simulink model "ex_2_20_1_simul"  (R2025a)
settings: Solver=VariableStepAuto  StartTime=0.0  StopTime=10.0  MaxStep=0.01  RelTol=1e-3
libraries: dspsrcs4 x1
settings Model: Creator=konstantin  LastModifiedBy=konstantin

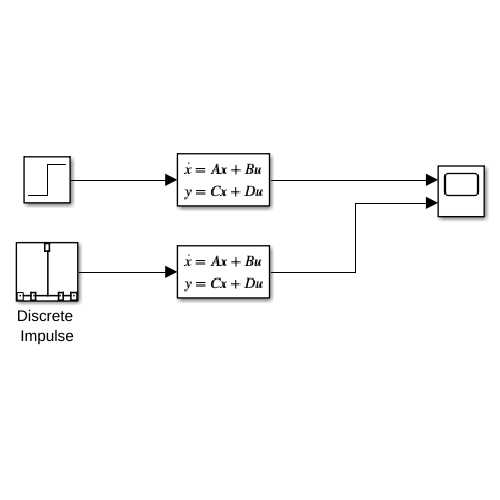
[thumbnail: Simulink's stored preview of the top-level diagram]
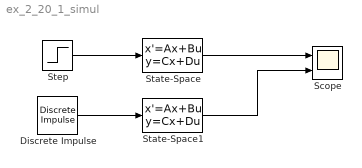
== system ex_2_20_1_simul ==
  Discrete Impulse : dspsrcs4/Discrete  Impulse  Delay=1  SampleTime=1  FrameSample=1  OutputFrames=off  dataType=double  isSigned=on  wordLen=16  udDataType=sfix(16)  fracBitsMode=Best precision  numFracBits=15  OutDataTypeStr=double  LastOutDataTypeStr=double
  Scope : Scope  NumInputPorts=2
      settings: ActiveDisplayYMinimum=-0.24999998857845496  ActiveDisplayYMaximum=2.2499998972060951
  State-Space : StateSpace  A=[-5, -6; 1, 0]  B=[1; 0]  C=[0, 12]  D=0  InitialCondition=0
  State-Space1 : StateSpace  A=[-5, -6; 1, 0]  B=[1; 0]  C=[0, 12]  D=0  InitialCondition=0
  Step : Step  SampleTime=0
  wires:
  Step/1 -> State-Space/1
  State-Space/1 -> Scope/1
  Discrete Impulse/1 -> State-Space1/1
  State-Space1/1 -> Scope/2
